simulink model "Linear_Model_Check_mks_4Nov_arbitaryinput"  (R2022b)
settings: Solver=VariableStepAuto  StartTime=0.0  StopTime=10000  FixedStep=0.5  RelTol=1e-6
settings Model: Creator=Mitarbeiter  LastModifiedBy=Mitarbeiter

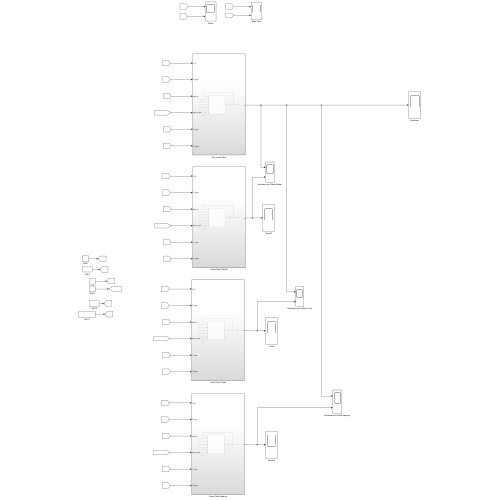
[thumbnail: Simulink's stored preview of the top-level diagram]
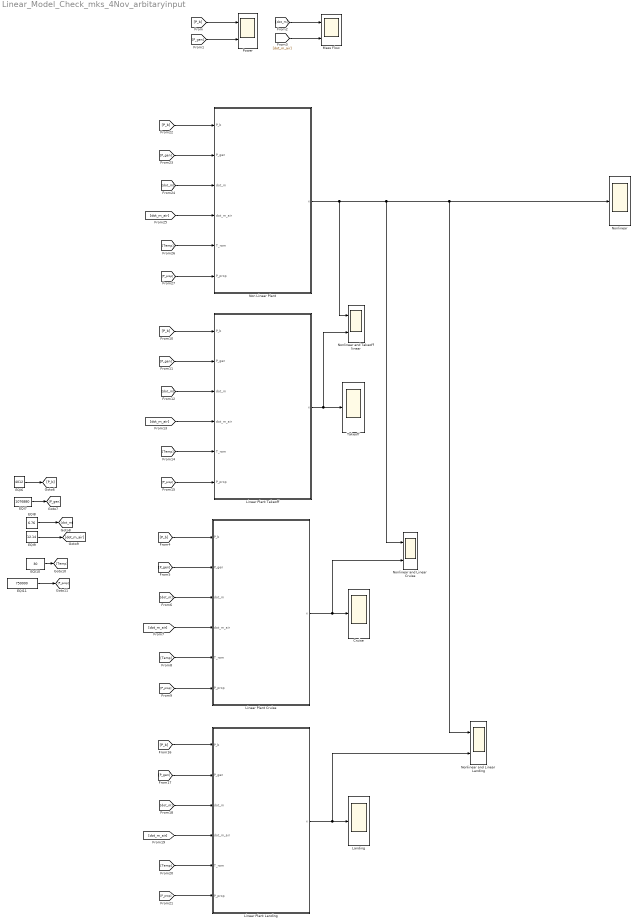
== system Linear_Model_Check_mks_4Nov_arbitaryinput ==
  Cruise : Scope
  EQI10 : Constant  Value=30
  EQI11 : Constant  Value=750000
  EQI6 : Constant  Value=4012  SampleTime=-1
  EQI7 : Constant  Value=1076880
  EQI8 : Constant  Value=6.76
  EQI9 : Constant  Value=12.14
  Landing : Scope
  Linear Plant Cruise : Subsystem
  Linear Plant Landing : Subsystem
  Linear Plant Takeoff : Subsystem
  Mass Flow : Scope  NumInputPorts=2
  Non Linear Plant : Subsystem
  Nonlinear : Scope
  Nonlinear and Linear Cruise : Scope  NumInputPorts=2
  Nonlinear and Linear Landing : Scope  NumInputPorts=2
  "Nonlinear and Takeoff linear " : Scope  NumInputPorts=2
  Power : Scope  NumInputPorts=2
  Takeoff : Scope
  wires:
  [P_b] -> Power/1
  [P_gen] -> Power/2
  [dot_m] -> Mass Flow/1
  [dot_m_air] -> Mass Flow/2
  EQI6/1 -> [P_b]
  EQI7/1 -> [P_gen]
  EQI8/1 -> [dot_m]
  EQI9/1 -> [dot_m_air]
  EQI10/1 -> [Temp]
  EQI11/1 -> [P_prop]
  [Temp] -> Linear Plant Takeoff/5(T_ram)
  [P_prop] -> Linear Plant Takeoff/6(P_prop)
  [dot_m_air] -> Linear Plant Takeoff/4(dot_m_air)
  [P_gen] -> Linear Plant Takeoff/2(P_gen)
  [P_b] -> Linear Plant Takeoff/1(P_b)
  Linear Plant Takeoff/1(x) -> Takeoff/1, "Nonlinear and Takeoff linear "/2
  [dot_m] -> Linear Plant Takeoff/3(dot_m)
  [P_b] -> Linear Plant Cruise/1(P_b)
  [dot_m] -> Linear Plant Cruise/3(dot_m)
  Linear Plant Cruise/1(x) -> Nonlinear and Linear Cruise/2, Cruise/1
  [Temp] -> Linear Plant Cruise/5(T_ram)
  [P_prop] -> Linear Plant Cruise/6(P_prop)
  [dot_m_air] -> Linear Plant Cruise/4(dot_m_air)
  [P_gen] -> Linear Plant Cruise/2(P_gen)
  [P_gen] -> Linear Plant Landing/2(P_gen)
  [dot_m_air] -> Linear Plant Landing/4(dot_m_air)
  [P_b] -> Linear Plant Landing/1(P_b)
  [P_prop] -> Linear Plant Landing/6(P_prop)
  [dot_m] -> Linear Plant Landing/3(dot_m)
  Linear Plant Landing/1(x) -> Nonlinear and Linear Landing/2, Landing/1
  [Temp] -> Linear Plant Landing/5(T_ram)
  [P_b] -> Non Linear Plant/1(P_b)
  [dot_m] -> Non Linear Plant/3(dot_m)
  Non Linear Plant/1(x) -> Nonlinear and Linear Cruise/1, Nonlinear and Linear Landing/1, Nonlinear/1, "Nonlinear and Takeoff linear "/1
  [Temp] -> Non Linear Plant/5(T_ram)
  [P_prop] -> Non Linear Plant/6(P_prop)
  [dot_m_air] -> Non Linear Plant/4(dot_m_air)
  [P_gen] -> Non Linear Plant/2(P_gen)

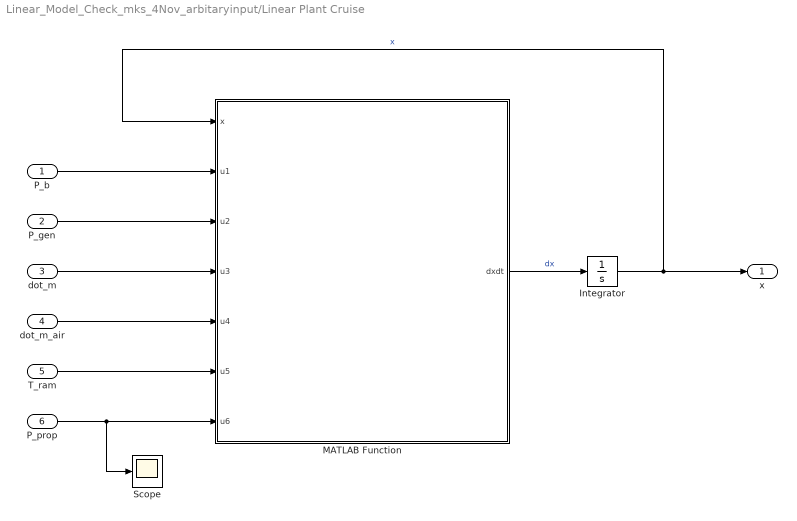
== system Linear_Model_Check_mks_4Nov_arbitaryinput/Linear Plant Cruise ==
  P_b : Inport
  P_gen : Inport  Port=2
  dot_m : Inport  Port=3
  dot_m_air : Inport  Port=4
  T_ram : Inport  Port=5
  P_prop : Inport  Port=6
  Integrator : Integrator  InitialCondition=[52814776030872794621339/2111078349043945281000; 104094200346052350023/4282106184673317000; 0.95; 7429519190417529794477/301582621291992183000; 14970426814841764289/611729454953331000; 62413813461003262061339/2111078349043945281000; 115709353125739950023/4282106184673317000; 1317031521595249/55809639171000; 192210910256741628225757/6125247032447703303000; 18157083865504564289/611729454953331000; 1317031521595249/55809639171000; 29037669531913/1240214203800; 1405698391771/60204573000];
  MATLAB Function : MATLAB Function  TreatAsAtomicUnit=on
  Scope : Scope
  x : Outport
  wires:
  MATLAB Function/1(dxdt) -> Integrator/1  "dx"
  Integrator/1 -> x/1, MATLAB Function/1(x)  "x"
  P_prop/1 -> Scope/1, MATLAB Function/7(u6)
  P_b/1 -> MATLAB Function/2(u1)
  P_gen/1 -> MATLAB Function/3(u2)
  dot_m/1 -> MATLAB Function/4(u3)
  dot_m_air/1 -> MATLAB Function/5(u4)
  T_ram/1 -> MATLAB Function/6(u5)

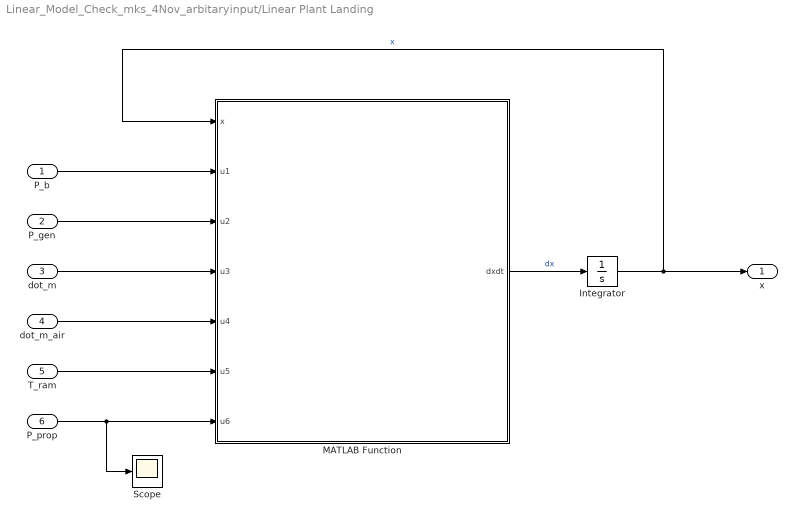
== system Linear_Model_Check_mks_4Nov_arbitaryinput/Linear Plant Landing ==
  P_b : Inport
  P_gen : Inport  Port=2
  dot_m : Inport  Port=3
  dot_m_air : Inport  Port=4
  T_ram : Inport  Port=5
  P_prop : Inport  Port=6
  Integrator : Integrator  InitialCondition=[93988057444394599308387229/4422589792359066198000000; 14175896344014406900981/690059259222822000000; 0.95; 642296550198010131218710603/30958128546513463386000000; 99794188918686328306867/4830414814559754000000; 748871653711516104483208603/30958128546513463386000000; 109523475430206270118867/4830414814559754000000; 114489338227757388521/5840888530302000000; 1232797079008717771442215271/48366943538186816802000000; 118698981952749594118867/4830414814559754000000; 114489338227757388521/5840888530302000000; 1053909433374709813/54082301206500000; 8752431102689/450060759000]
  MATLAB Function : MATLAB Function  TreatAsAtomicUnit=on
  Scope : Scope
  x : Outport
  wires:
  MATLAB Function/1(dxdt) -> Integrator/1  "dx"
  Integrator/1 -> x/1, MATLAB Function/1(x)  "x"
  P_prop/1 -> Scope/1, MATLAB Function/7(u6)
  P_b/1 -> MATLAB Function/2(u1)
  P_gen/1 -> MATLAB Function/3(u2)
  dot_m/1 -> MATLAB Function/4(u3)
  dot_m_air/1 -> MATLAB Function/5(u4)
  T_ram/1 -> MATLAB Function/6(u5)

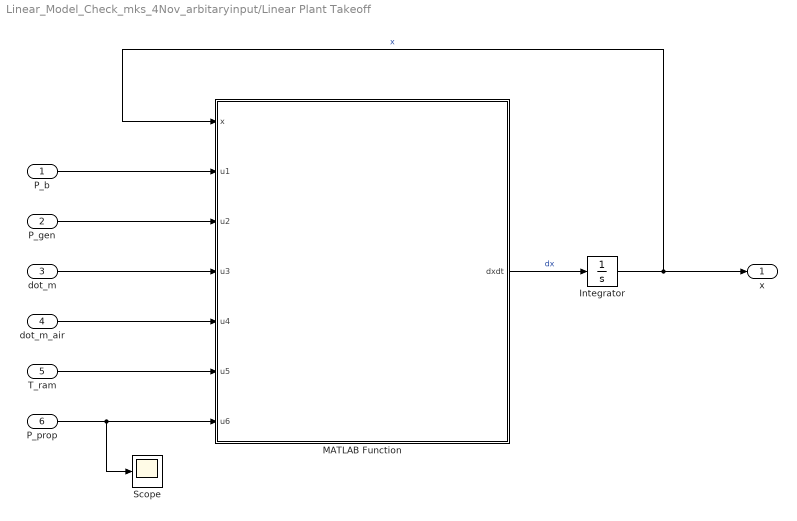
== system Linear_Model_Check_mks_4Nov_arbitaryinput/Linear Plant Takeoff ==
  P_b : Inport
  P_gen : Inport  Port=2
  dot_m : Inport  Port=3
  dot_m_air : Inport  Port=4
  T_ram : Inport  Port=5
  P_prop : Inport  Port=6
  Integrator : Integrator  InitialCondition=[20275100030210626643675627/393605954186145082200000; 2979945209973437579603/61414566107995800000; 0.95; 19353199461943751447675627/393605954186145082200000; 3002556108225437579603/61414566107995800000; 21715964372172979203125627/393605954186145082200000; 3222032306869374239603/61414566107995800000; 657622429946024881/14752478046600000; 37742600191627471661144839/614944050439361945400000; 3590589948376974239603/61414566107995800000; 657622429946024881/14752478046600000; 81610506679008893/1844059755825000; 9032287404091/204611346000]
  MATLAB Function : MATLAB Function  TreatAsAtomicUnit=on
  Scope : Scope
  x : Outport
  wires:
  MATLAB Function/1(dxdt) -> Integrator/1  "dx"
  Integrator/1 -> x/1, MATLAB Function/1(x)  "x"
  P_prop/1 -> Scope/1, MATLAB Function/7(u6)
  P_b/1 -> MATLAB Function/2(u1)
  P_gen/1 -> MATLAB Function/3(u2)
  dot_m/1 -> MATLAB Function/4(u3)
  dot_m_air/1 -> MATLAB Function/5(u4)
  T_ram/1 -> MATLAB Function/6(u5)

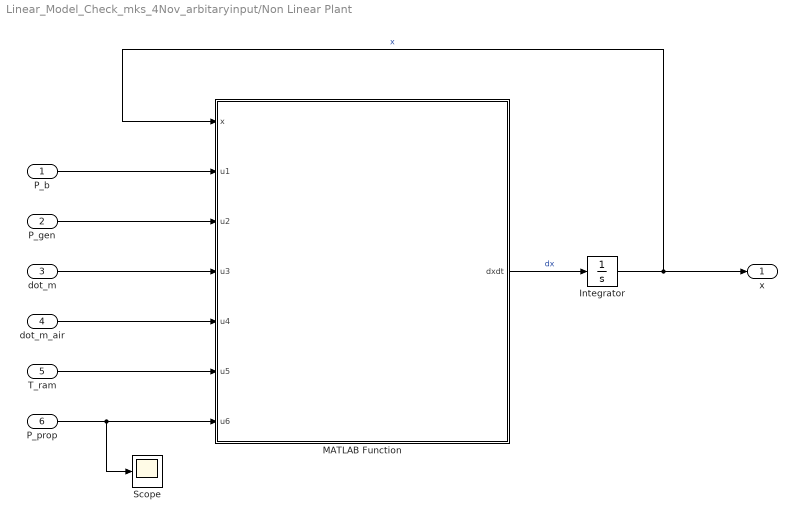
== system Linear_Model_Check_mks_4Nov_arbitaryinput/Non Linear Plant ==
  P_b : Inport
  P_gen : Inport  Port=2
  dot_m : Inport  Port=3
  dot_m_air : Inport  Port=4
  T_ram : Inport  Port=5
  P_prop : Inport  Port=6
  Integrator : Integrator  InitialCondition=[93988057444394599308387229/4422589792359066198000000; 14175896344014406900981/690059259222822000000; 0.95; 642296550198010131218710603/30958128546513463386000000; 99794188918686328306867/4830414814559754000000; 20; 748871653711516104483208603/30958128546513463386000000; 109523475430206270118867/4830414814559754000000; 20; 114489338227757388521/5840888530302000000; 20; 1232797079008717771442215271/48366943538186816802000000; 118698981952749594118867/4830414814559754000000; 114489338227757388521/5840888530302000000; 1053909433374709813/54082301206500000; 8752431102689/450060759000]
  MATLAB Function : MATLAB Function  TreatAsAtomicUnit=on
  Scope : Scope
  x : Outport
  wires:
  MATLAB Function/1(dxdt) -> Integrator/1  "dx"
  Integrator/1 -> x/1, MATLAB Function/1(x)  "x"
  P_prop/1 -> Scope/1, MATLAB Function/7(u6)
  P_b/1 -> MATLAB Function/2(u1)
  P_gen/1 -> MATLAB Function/3(u2)
  dot_m/1 -> MATLAB Function/4(u3)
  dot_m_air/1 -> MATLAB Function/5(u4)
  T_ram/1 -> MATLAB Function/6(u5)

== matlab function Linear_Model_Check_mks_4Nov_arbitaryinput/Linear Plant Cruise/MATLAB Function ==
  data: x input; dxdt output; u1 input; u2 input; u3 input; u4 input; u5 input; u6 input
function dxdt = fcn(x,u1,u2,u3,u4,u5,u6)

u = [u1;u2;u3;u4;u5;u6];
dxdt = aircraft_dynamics_linear_cruise(x,u);

== matlab function Linear_Model_Check_mks_4Nov_arbitaryinput/Linear Plant Landing/MATLAB Function ==
  data: x input; dxdt output; u1 input; u2 input; u3 input; u4 input; u5 input; u6 input
function dxdt = fcn(x,u1,u2,u3,u4,u5,u6)

u = [u1;u2;u3;u4;u5;u6];
dxdt = aircraft_dynamics_linear_landing(x,u);

== matlab function Linear_Model_Check_mks_4Nov_arbitaryinput/Linear Plant Takeoff/MATLAB Function ==
  data: x input; dxdt output; u1 input; u2 input; u3 input; u4 input; u5 input; u6 input
function dxdt = fcn(x,u1,u2,u3,u4,u5,u6)

u = [u1;u2;u3;u4;u5;u6];
dxdt = aircraft_dynamics_linear_takeoff(x,u);

== matlab function Linear_Model_Check_mks_4Nov_arbitaryinput/Non Linear Plant/MATLAB Function ==
  data: x input; dxdt output; u1 input; u2 input; u3 input; u4 input; u5 input; u6 input
function dxdt = fcn(x,u1,u2,u3,u4,u5,u6)

u = [u1;u2;u3;u4;u5;u6];
dxdt = aircraftDynamicsCT(x,u);
